simulink model "simple_dds"  (R2019b)
settings: Solver=FixedStepDiscrete  StartTime=0.0  StopTime=2e-6  FixedStep=1/128e6  RelTol=1e-3
InitFcn:
  | %axis_example_init
  | nco_setup
  | load('iq_bus_obj.mat')
libraries: hdlsllib x1
Description:
  | HDL model for RFSoC ADC/DAC IQ 8x8 interfacing with the mixer enabled
  | 
  | This model contains demonstrates how to interface to all 8 ADC and 8 DAC
  | channels for the RFSoC.
  | 
  | Please ensure that you run the initialization script to set the correct PLL clock rates.
settings Model: DataTypeOverride=Off  Creator=mfornero  LastModifiedBy=larry
settings SolverCC: AutoInsertRateTranBlk=on
settings DataIOCC: SaveOutput=off  SaveTime=off  ReturnWorkspaceOutputs=off
settings OptimizationCC: BlockReduction=off  ConditionallyExecuteInputs=off  DefaultParameterBehavior=Inlined  LifeSpan=inf
settings DebuggingCC: AlgebraicLoopMsg=error  SingleTaskRateTransMsg=error  PregeneratedLibrarySubsystemCodeDiagnostic=none  StrictBusMsg=ErrorOnBusTreatedAsVector  SFUnexpectedBacktrackingDiag=warning  SFNoUnconditionalDefaultTransitionDiag=warning  SFExecutionAtInitializationDiag=none  ArithmeticOperatorsInVariantConditions=warning
settings HardwareCC: ProdBitPerPointer=32  ProdBitPerSizeT=32  ProdBitPerPtrDiffT=32  ProdLargestAtomicFloat=None  ProdIntDivRoundTo=Undefined  ProdEndianess=Unspecified  ProdWordSize=32  ProdHWDeviceType=ASIC/FPGA->ASIC/FPGA  ProdEqTarget=off
settings SFSimCC: SimUseLocalCustomCode=off  CustomCodeUndefinedFunction=UseInterfaceOnly
settings RTWCC: RTWUseLocalCustomCode=off
settings CodeAppCC: StateflowObjectComments=on
settings GRTTargetCC: TargetLangStandard=C89/C90 (ANSI)
settings ConfigComp: CovMetricSettings=dw  CovHtmlReporting=on  CovSaveCumulativeToWorkspaceVar=on  CovSaveSingleToWorkspaceVar=on  CovExternalEMLEnable=off

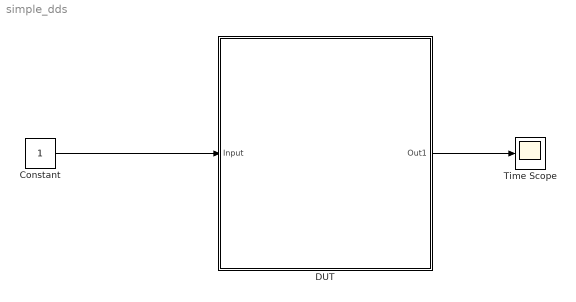
== system simple_dds ==
  Constant : Constant  OutDataTypeStr=boolean
  DUT : Subsystem
  Time Scope : Scope
  wires:
  DUT/1(Out1) -> Time Scope/1
  Constant/1 -> DUT/1(Input)

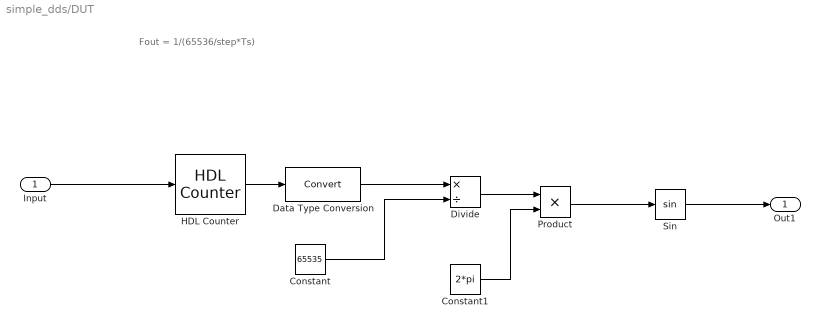
== system simple_dds/DUT ==
  note: Fout = 1/(65536/step*Ts)
  Input : Inport
  Constant : Constant  Value=65535  SampleTime=-1
  Constant1 : Constant  Value=2*pi  SampleTime=-1
  Data Type Conversion : DataTypeConversion
  Divide : Product  Inputs=*/
  HDL Counter : hdlsllib/Sources/HDL Counter  CountType=Free running  CountInit=0  CountStep=16383  CountMax=25  CountFromType=Initial value  CountFrom=0  CountResetPort=off  CountLoadPort=off  CountEnbPort=on  CountDirPort=off  CountDataType=Unsigned  CountWordLen=16  CountFracLen=0  CountSampTime=1
      settings: SourceProductName=Simulink
  Product : Product
  Sin : Trigonometry
  Out1 : Outport
  wires:
  HDL Counter/1 -> Data Type Conversion/1
  Constant/1 -> Divide/2
  Divide/1 -> Product/1
  Constant1/1 -> Product/2
  Product/1 -> Sin/1
  Sin/1 -> Out1/1
  Data Type Conversion/1 -> Divide/1
  Input/1 -> HDL Counter/1
